simulink model "Ecuacion_Diferenciales_Extrusora_de_Plastico_Ejercicio_7"  (R2017b)
settings: Solver=VariableStepAuto  StartTime=0.0  StopTime=1000  RelTol=1e-3
settings Model: Creator=Elmer  LastModifiedBy=Elmer

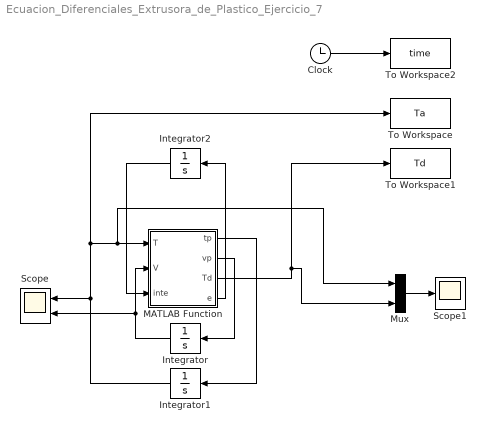
== system Ecuacion_Diferenciales_Extrusora_de_Plastico_Ejercicio_7 ==
  Clock : Clock
  Integrator : Integrator
  Integrator1 : Integrator
  Integrator2 : Integrator
  MATLAB Function : MATLAB Function  TreatAsAtomicUnit=on
  Mux : Mux  Inputs=2
  Scope : Scope  NumInputPorts=2
  Scope1 : Scope
  To Workspace : ToWorkspace  VariableName=Ta  SampleTime=-1
  To Workspace1 : ToWorkspace  VariableName=Td  SampleTime=-1
  To Workspace2 : ToWorkspace  VariableName=time  SampleTime=-1
  wires:
  MATLAB Function/2(vp) -> Integrator/1
  MATLAB Function/1(tp) -> Integrator1/1
  Integrator/1 -> Scope/2, MATLAB Function/2(V)
  Integrator1/1 -> MATLAB Function/1(T), Mux/1, To Workspace/1, Scope/1
  MATLAB Function/3(Td) -> To Workspace1/1, Mux/2
  Mux/1 -> Scope1/1
  Clock/1 -> To Workspace2/1
  MATLAB Function/4(e) -> Integrator2/1
  Integrator2/1 -> MATLAB Function/3(inte)

== matlab function Ecuacion_Diferenciales_Extrusora_de_Plastico_Ejercicio_7/MATLAB Function ==
  data: T input; tp output; V input; vp output; Td output; e output; inte input
function [tp,vp,Td,e]= fcn(T,V,inte)

h=133; Cp=1350; Ve=0.0207; R=1380; A=0.2;

a1=h*A/(R*Cp*Ve);
a2=1/(R*Cp*Ve);

%Controlador
%Kp=5;
%Td=120;
%e=Td-T;
%g=Kp*e;

%Controlador 2
Kp=400;
Td=120;
e=Td-T;
Ki=80;
g=Kp*e+Ki*inte;

tp=a1*T+V;
vp=a2*g;
